simulink model "ebike_01"  (Simulink 8.5)
settings: Solver=ode45  StartTime=0.0  StopTime=0.5  RelTol=1e-3
values from neighbouring files (symbols this model uses):
  A = 0.38    [run_sim.m]
  Cr = 0.003    [run_sim.m]
  Cw = 0.8    [run_sim.m]
  M_Bike = input('Enter the mass of Bike in Kilograms')    [run_sim.m]
  M_Driver = input('Enter the mass of Driver in kilograms' )    [run_sim.m]
libraries: simulink x3
settings Model: Creator=sabaribalu6691  LastModifiedBy=sabaribalu6691
settings DataIOCC: SignalLoggingSaveFormat=Dataset
settings OptimizationCC: ExpressionDepthLimit=128
settings DebuggingCC: UnderspecifiedInitializationDetection=Simplified  MergeDetectMultiDrivingBlocksExec=error  FcnCallInpInsideContextMsg=EnableAllAsError  StateNameClashWarn=none
settings GRTTargetCC: CombineOutputUpdateFcns=on  GRTInterface=off

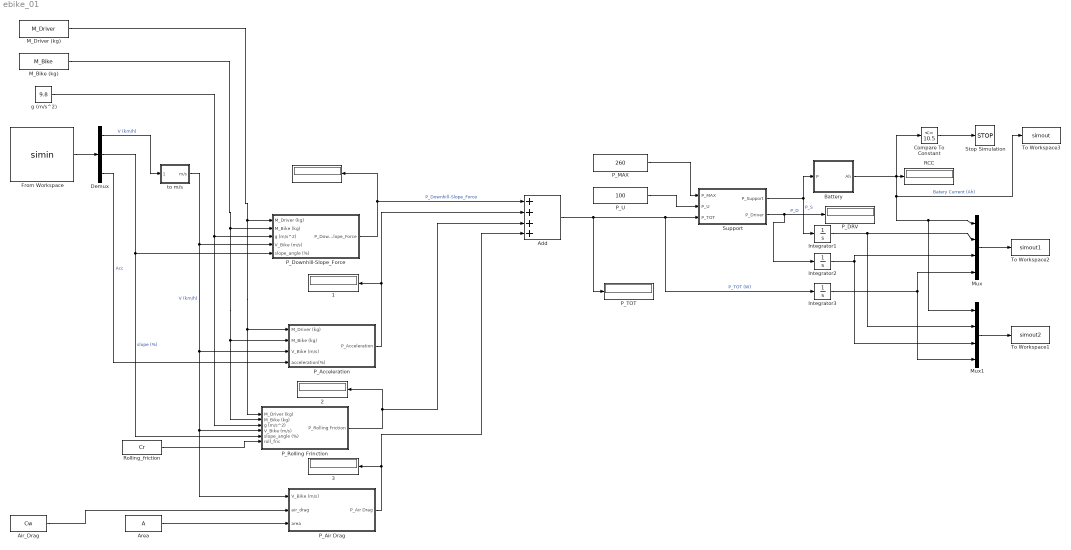
== system ebike_01 ==
     {,1..3} (4 alike) : Display
  " P_DRV" : Display
  " P_TOT" : Display
  Add : Sum  Inputs=++++
  Air_Drag : Constant  Value=Cw
  Area : Constant  Value=A
  Battery : Subsystem
  Compare To Constant : simulink/Logic and Bit Operations/Compare To Constant  relop=<=  const=10.5  OutDataTypeStr=boolean
  Demux : Demux  Outputs=3
  From Workspace : FromWorkspace  VariableName=simin  SampleTime=0  OutputAfterFinalValue=Holding final value
  Integrator1 : Integrator
  Integrator2 : Integrator
  Integrator3 : Integrator
  M_Bike (kg) : Constant  Value=M_Bike
  M_Driver (kg) : Constant  Value=M_Driver
  Mux : Mux
  Mux1 : Mux
  P_Acceleration : Subsystem
  P_Air Drag : Subsystem
  P_Downhill-Slope_Force : Subsystem
  P_MAX : Constant  Value=260
  P_Rolling Frinction : Subsystem
  P_U : Constant  Value=100
  RCC : Display
  Rolling_friction : Constant  Value=Cr
  Stop Simulation : Stop
  Support : Subsystem
  To Workspace1 : ToWorkspace  VariableName=simout2  SaveFormat=Structure With Time  SampleTime=-1
  To Workspace2 : ToWorkspace  VariableName=simout1  SaveFormat=Structure With Time  SampleTime=-1
  To Workspace3 : ToWorkspace  VariableName=simout  SaveFormat=Structure With Time  SampleTime=-1
  g (m/s^2) : Constant  Value=9.8
  to m/s : Subsystem
  wires:
  M_Driver (kg)/1 -> P_Rolling Frinction/1(M_Driver (kg)), P_Acceleration/1(M_Driver (kg)), P_Downhill-Slope_Force/1(M_Driver (kg))
  M_Bike (kg)/1 -> P_Rolling Frinction/2(M_Bike (kg)), P_Acceleration/2(M_Bike (kg)), P_Downhill-Slope_Force/2(M_Bike (kg))
  g (m/s^2)/1 -> P_Rolling Frinction/3(g (m/s^2)), P_Downhill-Slope_Force/3(g (m/s^2))
  From Workspace/1 -> Demux/1
  Demux/1 -> to m/s/1(km/h)  "V (km/h)"
  Demux/2 -> P_Rolling Frinction/5(slope_angle (%)), P_Downhill-Slope_Force/5(slope_angle (%))  "slope (%)"
  Demux/3 -> P_Acceleration/4(acceleration(%))  "Acc"
  Rolling_friction/1 -> P_Rolling Frinction/6(roll_fric)
  Air_Drag/1 -> P_Air Drag/2(air_drag)
  Area/1 -> P_Air Drag/3(area)
  P_Downhill-Slope_Force/1(P_Downhill-Slope_Force) -> Add/1, "   "/1  "P_Downhill-Slope_Force"
  Support/1(P_Support) -> Battery/1(P), Integrator1/1  "P_S"
  Support/2(P_Driver) -> Integrator2/1, " P_DRV"/1  "P_D"
  Battery/1(Ah) -> Compare To Constant/1, To Workspace3/1, Mux1/1, Mux/1, RCC/1  "Batery Current (Ah)"
  to m/s/1(m/s) -> P_Acceleration/3(V_Bike (m/s)), P_Air Drag/1(V_Bike (m/s)), P_Rolling Frinction/4(V_Bike (m/s)), P_Downhill-Slope_Force/4(V_Bike (m/s))  "V (km/h)"
  P_Acceleration/1(P_Acceleration) -> Add/2, "   1"/1
  P_Rolling Frinction/1(P_Rolling Friction) -> Add/3, "   2"/1
  P_Air Drag/1(P_Air Drag) -> Add/4, "   3"/1
  Add/1 -> Integrator3/1, Support/3(P_TOT), " P_TOT"/1  "P_TOT (W)"
  Mux/1 -> To Workspace2/1
  P_U/1 -> Support/2(P_U)
  P_MAX/1 -> Support/1(P_MAX)
  Mux1/1 -> To Workspace1/1
  Integrator1/1 -> Mux1/2, Mux/2
  Integrator2/1 -> Mux/3, Mux1/3
  Integrator3/1 -> Mux1/4, Mux/4
  Compare To Constant/1 -> Stop Simulation/1

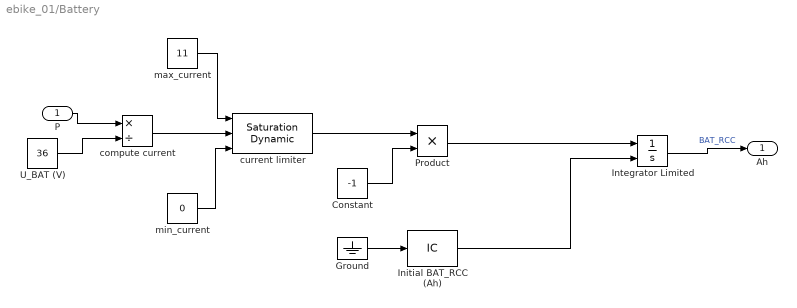
== system ebike_01/Battery ==
  P : Inport
  Constant : Constant  Value=-1
  Ground : Ground
  Initial BAT_RCC (Ah) : InitialCondition  Value=11
  Integrator Limited : Integrator  InitialConditionSource=external  LimitOutput=on  UpperSaturationLimit=13  LowerSaturationLimit=0
  Product : Product  RndMeth=Zero
  U_BAT (V) : Constant  Value=36
  compute current : Product  Inputs=*/
  current limiter : simulink/Discontinuities/Saturation Dynamic  OutMin=[]  OutMax=[]  OutDataTypeStr=Inherit: Same as second input  OutDataType=fixdt(1, 16)  OutScaling=2^-10  DoSatur=on
  max_current : Constant  Value=11
  min_current : Constant  Value=0
  Ah : Outport
  wires:
  Ground/1 -> Initial BAT_RCC (Ah)/1
  U_BAT (V)/1 -> compute current/2
  Constant/1 -> Product/2
  Product/1 -> Integrator Limited/1
  P/1 -> compute current/1
  Integrator Limited/1 -> Ah/1  "BAT_RCC"
  current limiter/1 -> Product/1
  compute current/1 -> current limiter/2
  max_current/1 -> current limiter/1
  min_current/1 -> current limiter/3
  Initial BAT_RCC (Ah)/1 -> Integrator Limited/2

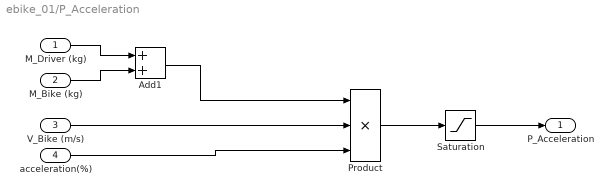
== system ebike_01/P_Acceleration ==
  M_Driver (kg) : Inport
  M_Bike (kg) : Inport  Port=2
  V_Bike (m/s) : Inport  Port=3
  acceleration(%) : Inport  Port=4
  Add1 : Sum
  Product : Product  Inputs=3  RndMeth=Zero
  Saturation : Saturate  UpperLimit=10000  LowerLimit=0
  P_Acceleration : Outport
  wires:
  Add1/1 -> Product/1
  M_Driver (kg)/1 -> Add1/1
  M_Bike (kg)/1 -> Add1/2
  V_Bike (m/s)/1 -> Product/2
  acceleration(%)/1 -> Product/3
  Product/1 -> Saturation/1
  Saturation/1 -> P_Acceleration/1

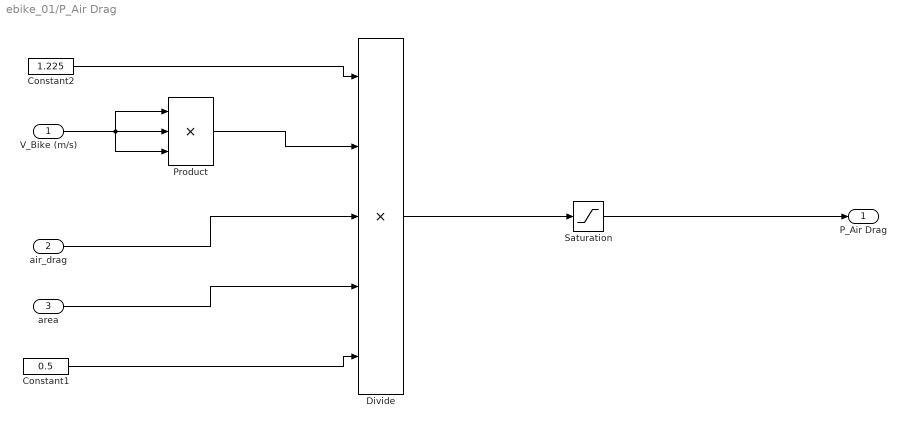
== system ebike_01/P_Air Drag ==
  V_Bike (m/s) : Inport
  air_drag : Inport  Port=2
  area : Inport  Port=3
  Constant1 : Constant  Value=0.5
  Constant2 : Constant  Value=1.225
  Divide : Product  Inputs=*****
  Product : Product  Inputs=3  RndMeth=Zero
  Saturation : Saturate  UpperLimit=10000  LowerLimit=0
  P_Air Drag : Outport
  wires:
  Saturation/1 -> P_Air Drag/1
  Constant2/1 -> Divide/1
  Divide/1 -> Saturation/1
  air_drag/1 -> Divide/3
  area/1 -> Divide/4
  Constant1/1 -> Divide/5
  V_Bike (m/s)/1 -> Product/3, Product/2, Product/1
  Product/1 -> Divide/2

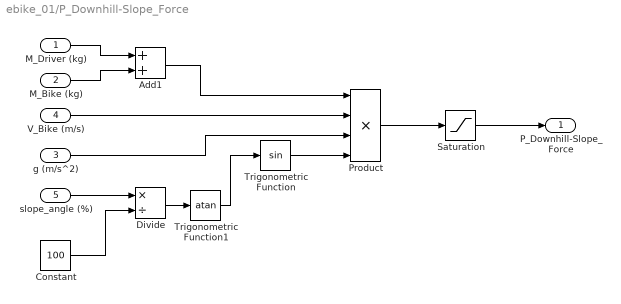
== system ebike_01/P_Downhill-Slope_Force ==
  M_Driver (kg) : Inport
  M_Bike (kg) : Inport  Port=2
  g (m/s^2) : Inport  Port=3
  V_Bike (m/s) : Inport  Port=4
  slope_angle (%) : Inport  Port=5
  Add1 : Sum
  Constant : Constant  Value=100
  Divide : Product  Inputs=*/
  Product : Product  Inputs=4  RndMeth=Zero
  Saturation : Saturate  UpperLimit=10000  LowerLimit=0
  Trigonometric Function : Trigonometry
  Trigonometric Function1 : Trigonometry  Operator=atan
  P_Downhill-Slope_Force : Outport
  wires:
  Add1/1 -> Product/1
  M_Driver (kg)/1 -> Add1/1
  M_Bike (kg)/1 -> Add1/2
  V_Bike (m/s)/1 -> Product/2
  g (m/s^2)/1 -> Product/3
  Trigonometric Function/1 -> Product/4
  Trigonometric Function1/1 -> Trigonometric Function/1
  slope_angle (%)/1 -> Divide/1
  Divide/1 -> Trigonometric Function1/1
  Constant/1 -> Divide/2
  Product/1 -> Saturation/1
  Saturation/1 -> P_Downhill-Slope_Force/1

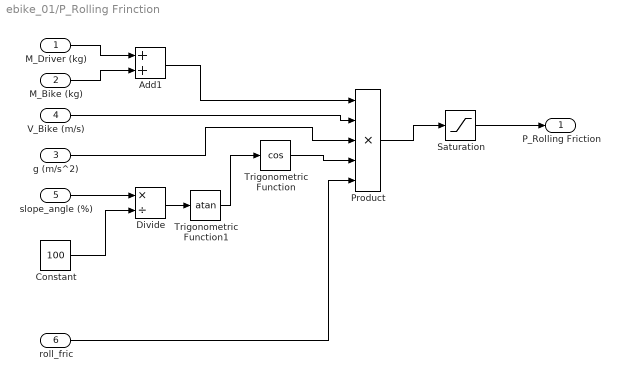
== system ebike_01/P_Rolling Frinction ==
  M_Driver (kg) : Inport
  M_Bike (kg) : Inport  Port=2
  g (m/s^2) : Inport  Port=3
  V_Bike (m/s) : Inport  Port=4
  slope_angle (%) : Inport  Port=5
  roll_fric : Inport  Port=6
  Add1 : Sum
  Constant : Constant  Value=100
  Divide : Product  Inputs=*/
  Product : Product  Inputs=5  RndMeth=Zero
  Saturation : Saturate  UpperLimit=10000  LowerLimit=0
  Trigonometric Function : Trigonometry  Operator=cos
  Trigonometric Function1 : Trigonometry  Operator=atan
  P_Rolling Friction : Outport
  wires:
  Add1/1 -> Product/1
  M_Driver (kg)/1 -> Add1/1
  M_Bike (kg)/1 -> Add1/2
  V_Bike (m/s)/1 -> Product/2
  g (m/s^2)/1 -> Product/3
  Trigonometric Function/1 -> Product/4
  Trigonometric Function1/1 -> Trigonometric Function/1
  slope_angle (%)/1 -> Divide/1
  Divide/1 -> Trigonometric Function1/1
  Constant/1 -> Divide/2
  Product/1 -> Saturation/1
  Saturation/1 -> P_Rolling Friction/1
  roll_fric/1 -> Product/5

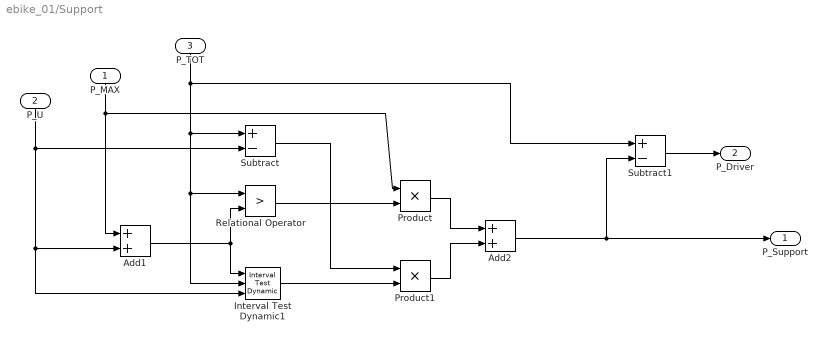
== system ebike_01/Support ==
  P_MAX : Inport
  P_U : Inport  Port=2
  P_TOT : Inport  Port=3
  Add1 : Sum
  Add2 : Sum
  Interval Test Dynamic1 : simulink/Logic and Bit Operations/Interval Test Dynamic  IntervalClosedRight=on  IntervalClosedLeft=on  OutDataTypeStr=uint8
  Product : Product  RndMeth=Zero
  Product1 : Product  RndMeth=Zero
  Relational Operator : RelationalOperator  Operator=>  OutDataTypeStr=boolean
  Subtract : Sum  Inputs=+-
  Subtract1 : Sum  Inputs=+-
  P_Support : Outport
  P_Driver : Outport  Port=2
  wires:
  Add1/1 -> Interval Test Dynamic1/1, Relational Operator/2
  P_TOT/1 -> Subtract1/1, Subtract/1, Interval Test Dynamic1/2, Relational Operator/1
  P_U/1 -> Subtract/2, Interval Test Dynamic1/3, Add1/2
  P_MAX/1 -> Product/1, Add1/1
  Relational Operator/1 -> Product/2
  Subtract/1 -> Product1/1
  Interval Test Dynamic1/1 -> Product1/2
  Product/1 -> Add2/1
  Product1/1 -> Add2/2
  Add2/1 -> Subtract1/2, P_Support/1
  Subtract1/1 -> P_Driver/1

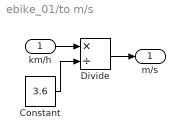
== system ebike_01/to m/s ==
  km/h : Inport
  Constant : Constant  Value=3.6
  Divide : Product  Inputs=*/
  m/s : Outport
  wires:
  Constant/1 -> Divide/2
  km/h/1 -> Divide/1
  Divide/1 -> m/s/1
